simulink subsystem "LeastCov_v1_adaptiveAlgorithm"  (R2022a)
settings: Solver=VariableStepAuto  StartTime=0.0  StopTime=10.0  RelTol=1e-3
libraries: simulink x2
settings Model: Creator=targi  LastModifiedBy=targi

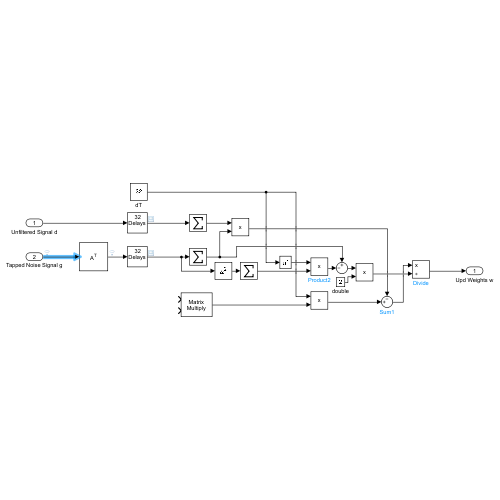
[thumbnail: Simulink's stored preview of the top-level diagram]
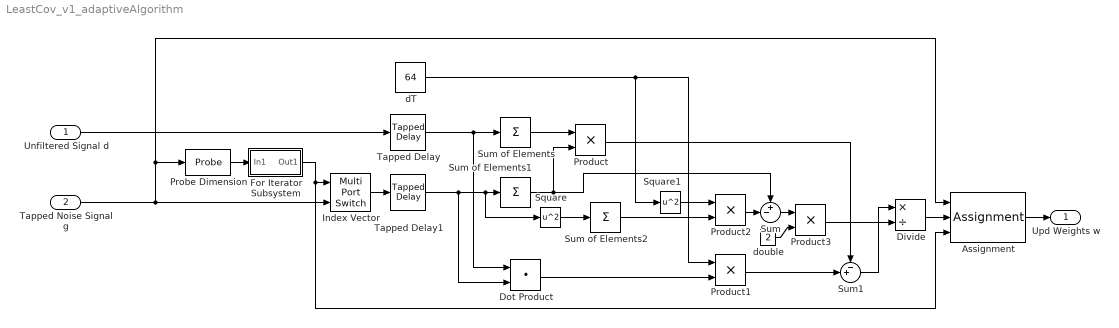
== system LeastCov_v1_adaptiveAlgorithm ==
  Unfiltered Signal d : Inport
  Tapped Noise Signal g : Inport  Port=2
  Assignment : Assignment  DiagnosticForDimensions=Warning  IndexOptions=Index vector (port)  Indices=1  OutputSizes=1
  Divide : Product  Inputs=*/
  Dot Product : DotProduct  OutDataTypeStr=Inherit: Inherit via internal rule
  For Iterator Subsystem : Subsystem  TreatAsAtomicUnit=on
  Index Vector : MultiPortSwitch  Inputs=1  SaturateOnIntegerOverflow=off  InputSameDT=off
  Probe Dimension : Probe  ProbeSampleTime=off  ProbeComplexSignal=off
  Product{,1..3} (4 alike) : Product
  Square : Math  Operator=square
  Square1 : Math  Operator=square
  Sum : Sum  Inputs=+-|
  Sum of Elements : Sum  Inputs=+
  Sum of Elements1 : Sum  Inputs=+
  Sum of Elements2 : Sum  Inputs=+
  Sum1 : Sum  Inputs=-+|
  Tapped Delay : simulink/Discrete/Tapped Delay  vinit=0.0  samptime=-1  NumDelays=64  DelayOrder=Oldest  includeCurrent=off
  Tapped Delay1 : simulink/Discrete/Tapped Delay  vinit=0.0  samptime=-1  NumDelays=64  DelayOrder=Oldest  includeCurrent=off
  dT : Constant  Value=64
  double : Constant  Value=2
  Upd Weights w : Outport
  wires:
  Unfiltered Signal d/1 -> Tapped Delay/1
  Tapped Delay/1 -> Sum of Elements/1, Dot Product/1
  Tapped Delay1/1 -> Square/1, Sum of Elements1/1, Dot Product/2
  Sum of Elements/1 -> Product/1
  Sum of Elements1/1 -> Sum/1, Product/2
  Square/1 -> Sum of Elements2/1
  Dot Product/1 -> Product1/2
  dT/1 -> Product1/1, Square1/1
  Sum of Elements2/1 -> Product2/2
  Square1/1 -> Product2/1
  Product2/1 -> Sum/2
  Product1/1 -> Sum1/2
  Product/1 -> Sum1/1
  Sum/1 -> Product3/1
  double/1 -> Product3/2
  Product3/1 -> Divide/2
  Sum1/1 -> Divide/1
  Index Vector/1 -> Tapped Delay1/1
  Tapped Noise Signal g/1 -> Index Vector/2, Probe Dimension/1, Assignment/1
  For Iterator Subsystem/1(Out1) -> Assignment/3, Index Vector/1
  Divide/1 -> Assignment/2
  Assignment/1 -> Upd Weights w/1
  Probe Dimension/1 -> For Iterator Subsystem/1(In1)

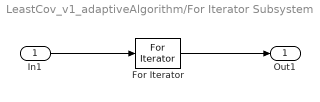
== system LeastCov_v1_adaptiveAlgorithm/For Iterator Subsystem ==
  In1 : Inport
  For Iterator : ForIterator  IterationSource=external
  Out1 : Outport
  wires:
  For Iterator/1 -> Out1/1
  In1/1 -> For Iterator/1
